simulink model "r_128w_8k_1a_16x_r431"  (R2012b)
settings: Solver=FixedStepDiscrete  SolverMode=SingleTasking  StartTime=0.0  StopTime=5000  RelTol=1e-3
undefined symbols (not defined in the file): Down, pfb_coeff_gen_calc, Up
libraries: xbsIndex_r4 x9410, casper_library_misc x257, casper_library_delays x92, xps_library x57, simulink x16, dspsigops x12, casper_library_flow_control x8, xbsReplacements_r4 x4, casper_library_multipliers x4, casper_library_scopes x2, casper_library_ffts_twiddle x2
(part 66 of 125)

== system r_128w_8k_1a_16x_r431/fft_wideband_real1/fft_direct/butterfly1_0/twiddle_general_dsp48e/coeff_gen ==
  rst : Inport
  Counter : xbsIndex_r4/Counter  cnt_type=Free Running  cnt_to=Inf  operation=Up  start_count=0  cnt_by_val=1  arith_type=Unsigned  n_bits=12  bin_pt=0  load_pin=off  rst=on  en=off  explicit_period=on  period=1  dbl_ovrd=off  use_behavioral_HDL=off  implementation=Fabric  block_type=counter
  ROM : xbsIndex_r4/ROM  depth=4096  initVector="[1                                      1                                      1                                      1                                      1                                      1                     0.9999847412109375                     0.9999847412109375                     0.9999847412109375                      0.999969482421875                      0.999969482421875                      0.999969482421875                     0.9999542236328125                     0.9999542236328125                       0.99993896484375                       0.99993896484375                     0.9999237060546875                      0.999908447265625                      0.999908447265625                     0.9998931884765625                        0.9998779296875                     0.9998626708984375                     0.9998626708984375                      0.999847412109375                     0.9998321533203125                       0.99981689453125                     0.9998016357421875                      0.999786376953125                     0.9997711181640625                         0.999755859375                     0.9997406005859375                     0.9997100830078125                       0.99969482421875                     0.9996795654296875                      0.999664306640625                        0.9996337890625                     0.9996185302734375                      0.999603271484375                       0.99957275390625                     0.9995574951171875                     0.9995269775390625                          0.99951171875                      0.999481201171875                       0.99945068359375                     0.9994354248046875                     0.9994049072265625                     0.9993743896484375                     0.9993438720703125                       0.99932861328125                      0.999298095703125                         0.999267578125                      0.999237060546875                       0.99920654296875                      0.999176025390625                        0.9991455078125                      0.999114990234375                       0.99908447265625                     0.9990386962890625                     0.9990081787109375                     0.9989776611328125                     0.9989471435546875                        0.9989013671875                      0.998870849609375                       0.99884033203125                     0.9987945556640625                     0.9987640380859375                       0.99871826171875                     0.9986724853515625                     0.9986419677734375                       0.99859619140625                      0.998565673828125                     0.9985198974609375                       0.99847412109375                     0.9984283447265625                      0.998382568359375                       0.99835205078125                     0.9983062744140625                      0.998260498046875                     0.9982147216796875                        0.9981689453125                     0.9981231689453125                      0.998077392578125                      0.998016357421875                     0.9979705810546875                        0.9979248046875                     0.9978790283203125                     0.9978179931640625                      0.997772216796875                     0.9977264404296875                     0.9976654052734375                       0.99761962890625                          0.99755859375                     0.9975128173828125                     0.9974517822265625                      0.997406005859375                      0.997344970703125                      0.997283935546875                     0.9972381591796875                     0.9971771240234375                     0.9971160888671875                     0.9970550537109375                     0.9969940185546875                        0.9969482421875 ...(+155708 chars)]"  distributed_mem=Block RAM  rst=off  init_reg=0  en=off  latency=2  gui_display_data_type=Fixed-point  arith_type="Signed  (2's comp)"  n_bits=18  bin_pt=16  preci_type=Single  exp_width=8  frac_width=24  dbl_ovrd=off  optimize=Area  use_rpm=on  block_type=sprom
  ROM1 : xbsIndex_r4/ROM  depth=4096  initVector="[0                     -0.000762939453125                    -0.0015411376953125                    -0.0023040771484375                    -0.0030670166015625                    -0.0038299560546875                     -0.004608154296875                         -0.00537109375                     -0.006134033203125                      -0.00689697265625                    -0.0076751708984375                    -0.0084381103515625                    -0.0092010498046875                    -0.0099639892578125                          -0.0107421875                     -0.011505126953125                      -0.01226806640625                     -0.013031005859375                    -0.0138092041015625                    -0.0145721435546875                    -0.0153350830078125                         -0.01611328125                     -0.016876220703125                      -0.01763916015625                     -0.018402099609375                    -0.0191802978515625                    -0.0199432373046875                    -0.0207061767578125                    -0.0214691162109375                     -0.022247314453125                      -0.02301025390625                     -0.023773193359375                       -0.0245361328125                    -0.0253143310546875                    -0.0260772705078125                    -0.0268402099609375                    -0.0276031494140625                      -0.02838134765625                     -0.029144287109375                       -0.0299072265625                     -0.030670166015625                    -0.0314483642578125                    -0.0322113037109375                    -0.0329742431640625                    -0.0337371826171875                    -0.0345001220703125                       -0.0352783203125                     -0.036041259765625                      -0.03680419921875                     -0.037567138671875                    -0.0383453369140625                    -0.0391082763671875                    -0.0398712158203125                    -0.0406341552734375                     -0.041412353515625                      -0.04217529296875                     -0.042938232421875                        -0.043701171875                     -0.044464111328125                    -0.0452423095703125                    -0.0460052490234375                    -0.0467681884765625                    -0.0475311279296875                    -0.0482940673828125                        -0.049072265625                     -0.049835205078125                      -0.05059814453125                     -0.051361083984375                    -0.0521392822265625                    -0.0529022216796875                    -0.0536651611328125                    -0.0544281005859375                    -0.0551910400390625                    -0.0559539794921875                     -0.056732177734375                       -0.0574951171875                     -0.058258056640625                      -0.05902099609375                     -0.059783935546875                    -0.0605621337890625                    -0.0613250732421875                    -0.0620880126953125                    -0.0628509521484375                    -0.0636138916015625                    -0.0643768310546875                     -0.065155029296875                         -0.06591796875                     -0.066680908203125                      -0.06744384765625                     -0.068206787109375                       -0.0689697265625                     -0.069732666015625                    -0.0705108642578125                    -0.0712738037109375                    -0.0720367431640625                    -0.0727996826171875                    -0.0735626220703125                    -0.0743255615234375                    -0.0750885009765625                      -0.07586669921875                     -0.076629638671875                        -0.077392578125                     -0.078155517578125 ...(+155708 chars)]"  distributed_mem=Block RAM  rst=off  init_reg=0  en=off  latency=2  gui_display_data_type=Fixed-point  arith_type="Signed  (2's comp)"  n_bits=18  bin_pt=16  preci_type=Single  exp_width=8  frac_width=24  dbl_ovrd=off  optimize=Area  use_rpm=on  block_type=sprom
  Slice : xbsIndex_r4/Slice  nbits=12  boolean_output=off  mode=Upper Bit Location + Width  bit1=0  base1=MSB of Input  bit0=0  base0=LSB of Input  dbl_ovrd=off  block_type=slice
  ri_to_c : casper_library_misc/ri_to_c
  w : Outport
  wires:
  ri_to_c/1 -> w/1
  rst/1 -> Counter/1
  Counter/1 -> Slice/1
  Slice/1 -> ROM/1, ROM1/1
  ROM/1 -> ri_to_c/1
  ROM1/1 -> ri_to_c/2
